simulink model "Lab4M"  (Simulink 5.0)
settings: Solver=ode45  StartTime=0.0  StopTime=1  RelTol=1e-3
libraries: simulink x5
settings Model: LastModifiedBy=Blue Phoenix

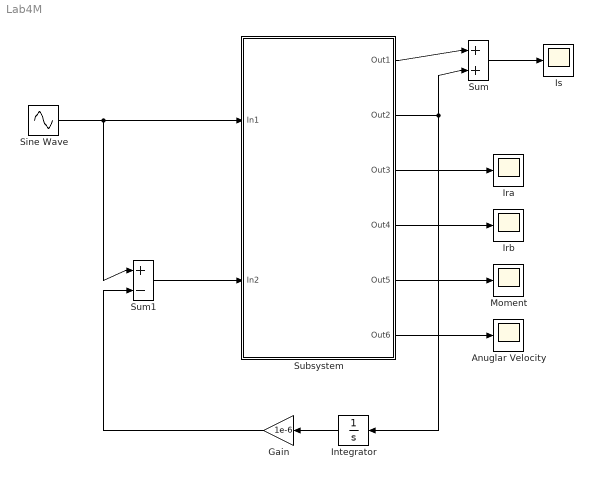
== system Lab4M ==
  Anuglar Velocity : Scope
      settings: SaveName=ScopeData5
  Gain : Gain  Orientation=left  Gain=1e-6  SaturateOnIntegerOverflow=on
  Integrator : Integrator  Orientation=left
  Ira : Scope
      settings: SaveName=ScopeData2
  Irb : Scope
      settings: SaveName=ScopeData3
  Is : Scope
  Moment : Scope
      settings: SaveName=ScopeData4
  Sine Wave : Sin  Amplitude=311  Frequency=314  SampleTime=0
  Subsystem : Subsystem
  Sum : Sum  Inputs=|++  SaturateOnIntegerOverflow=on
  Sum1 : Sum  Inputs=|+-  SaturateOnIntegerOverflow=on
  wires:
  Sine Wave/1 -> Subsystem/1(In1), Sum1/1
  Sum/1 -> Is/1
  Subsystem/1(Out1) -> Sum/1
  Subsystem/2(Out2) -> Sum/2, Integrator/1
  Subsystem/3(Out3) -> Ira/1
  Subsystem/4(Out4) -> Irb/1
  Subsystem/5(Out5) -> Moment/1
  Subsystem/6(Out6) -> Anuglar Velocity/1
  Sum1/1 -> Subsystem/2(In2)
  Integrator/1 -> Gain/1
  Gain/1 -> Sum1/2

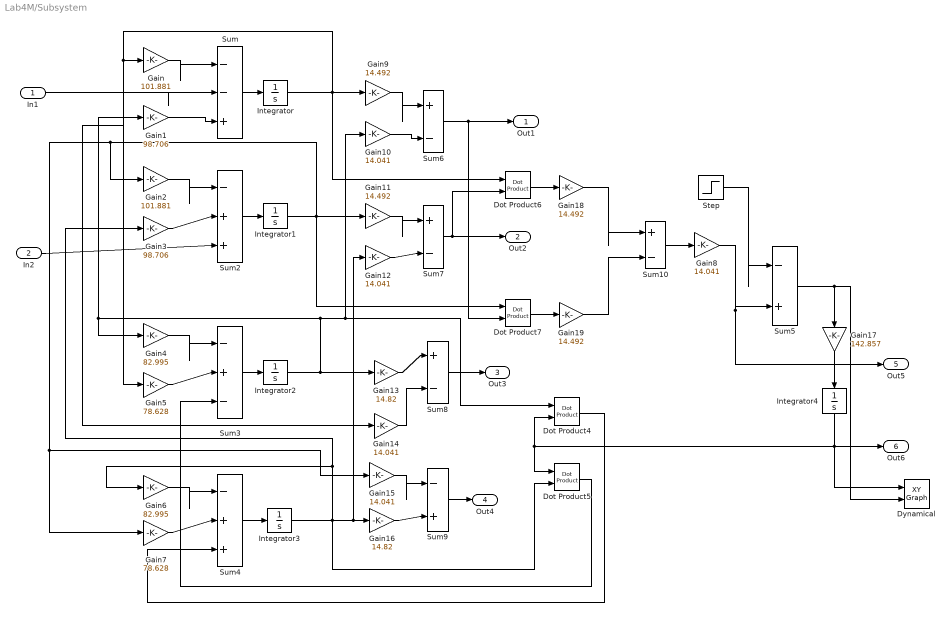
== system Lab4M/Subsystem ==
  In1 : Inport
  In2 : Inport  Port=2
  Dot Product{4..7} (4 alike) : simulink/Math Operations/Dot Product
  Dynamical : simulink/Sinks/XY Graph  xmin=-10  xmax=320  ymin=-5  ymax=5  st=-1
  Gain : Gain  Gain=101.881  ShowAdditionalParam=on  SaturateOnIntegerOverflow=on
  Gain1 : Gain  Gain=98.706  SaturateOnIntegerOverflow=on
  Gain{8,10,12,14..15} (5 alike) : Gain  Gain=14.041  SaturateOnIntegerOverflow=on
  Gain{9,11,18..19} (4 alike) : Gain  Gain=14.492  SaturateOnIntegerOverflow=on
  Gain13 : Gain  Gain=14.82  SaturateOnIntegerOverflow=on
  Gain16 : Gain  Gain=14.82  SaturateOnIntegerOverflow=on
  Gain17 : Gain  Orientation=down  Gain=142.857  ShowAdditionalParam=on  SaturateOnIntegerOverflow=on
  Gain2 : Gain  Gain=101.881  SaturateOnIntegerOverflow=on
  Gain3 : Gain  Gain=98.706  SaturateOnIntegerOverflow=on
  Gain4 : Gain  Gain=82.995  SaturateOnIntegerOverflow=on
  Gain5 : Gain  Gain=78.628  SaturateOnIntegerOverflow=on
  Gain6 : Gain  Gain=82.995  SaturateOnIntegerOverflow=on
  Gain7 : Gain  Gain=78.628  SaturateOnIntegerOverflow=on
  Integrator{,1..3} (4 alike) : Integrator
  Integrator4 : Integrator  Orientation=down
  Step : Step  Time=0  After=2.3  SampleTime=0
  Sum : Sum  Inputs=|--+  ShowAdditionalParam=on  SaturateOnIntegerOverflow=on
  Sum{6..8,10} (4 alike) : Sum  Inputs=|+-  ShowAdditionalParam=on  SaturateOnIntegerOverflow=on
  Sum2 : Sum  Inputs=|-++  ShowAdditionalParam=on  SaturateOnIntegerOverflow=on
  Sum3 : Sum  Inputs=|-+-  ShowAdditionalParam=on  SaturateOnIntegerOverflow=on
  Sum4 : Sum  Inputs=|-++  ShowAdditionalParam=on  SaturateOnIntegerOverflow=on
  Sum5 : Sum  Inputs=|-+  ShowAdditionalParam=on  SaturateOnIntegerOverflow=on
  Sum9 : Sum  Inputs=|-+  ShowAdditionalParam=on  SaturateOnIntegerOverflow=on
  Out1 : Outport
  Out2 : Outport  Port=2
  Out3 : Outport  Port=3
  Out4 : Outport  Port=4
  Out5 : Outport  Port=5
  Out6 : Outport  Port=6
  wires:
  Sum4/1 -> Integrator3/1
  Sum3/1 -> Integrator2/1
  Sum2/1 -> Integrator1/1
  Sum/1 -> Integrator/1
  Integrator1/1 -> Dot Product7/1, Gain2/1, Gain7/1, Gain15/1, Gain11/1
  Integrator2/1 -> Gain1/1, Gain4/1, Gain10/1, Dot Product4/1, Gain13/1
  Integrator/1 -> Gain/1, Gain5/1, Gain14/1, Dot Product6/1, Gain9/1
  Integrator3/1 -> Gain6/1, Gain3/1, Dot Product5/2, Gain16/1, Gain12/1
  Sum10/1 -> Gain8/1
  Sum6/1 -> Dot Product7/2, Out1/1
  Step/1 -> Sum5/1
  Gain8/1 -> Sum5/2, Out5/1
  Gain17/1 -> Integrator4/1
  Sum5/1 -> Gain17/1, Dynamical/2
  Integrator4/1 -> Dot Product4/2, Dot Product5/1, Out6/1, Dynamical/1
  Gain/1 -> Sum/1
  Gain4/1 -> Sum3/1
  Gain2/1 -> Sum2/1
  Gain1/1 -> Sum/3
  In2/1 -> Sum2/3
  Gain6/1 -> Sum4/1
  Gain7/1 -> Sum4/2
  Dot Product4/1 -> Sum4/3
  Dot Product5/1 -> Sum3/3
  Gain5/1 -> Sum3/2
  Gain9/1 -> Sum6/1
  Gain10/1 -> Sum6/2
  Gain11/1 -> Sum7/1
  Gain12/1 -> Sum7/2
  Gain13/1 -> Sum8/1
  Gain14/1 -> Sum8/2
  Gain16/1 -> Sum9/2
  Gain15/1 -> Sum9/1
  In1/1 -> Sum/2
  Gain3/1 -> Sum2/2
  Sum7/1 -> Dot Product6/2, Out2/1
  Sum8/1 -> Out3/1
  Sum9/1 -> Out4/1
  Dot Product6/1 -> Gain18/1
  Dot Product7/1 -> Gain19/1
  Gain18/1 -> Sum10/1
  Gain19/1 -> Sum10/2
